simulink model "systemmain"  (R2017b)
settings: Solver=VariableStepAuto  StartTime=0.0  StopTime=20  RelTol=1e-3
values from neighbouring files (symbols this model uses):
  Kd_alt = 0    [Controller_Tuning.m]
  Kd_pitch = 0    [Controller_Tuning.m]
  Kd_roll = 0    [Controller_Tuning.m]
  Kd_yaw = 0    [Controller_Tuning.m]
  Ki_alt = 0    [Controller_Tuning.m]
  Ki_pitch = 1    [Controller_Tuning.m]
  Ki_roll = 1    [Controller_Tuning.m]
  Ki_yaw = 1    [Controller_Tuning.m]
  Kp_alt = 1    [Controller_Tuning.m]
  Kp_pitch = 1    [Controller_Tuning.m]
  Kp_roll = 1    [Controller_Tuning.m]
  Kp_yaw = 1    [Controller_Tuning.m]
  phiaccinitial = 0    [startup.m]
  phiinitial = 0    [startup.m]
  phivelinitial = 0    [startup.m]
  psiaccinitial = 0    [startup.m]
  psiinitial = 0    [startup.m]
  psivelinitial = 0    [startup.m]
  thetaaccinitial = 0    [startup.m]
  thetainitial = 0    [startup.m]
  thetavelinitial = 0    [startup.m]
  xaccinitial = 0    [startup.m]
  xinitial = 0    [startup.m]
  xvelinitial = 0    [startup.m]
  yaccinitial = 0    [startup.m]
  yinitial = 0    [startup.m]
  yvelinitial = 0    [startup.m]
  zaccinitial = 0    [startup.m]
  zinitial = 10    [startup.m]
  zvelinitial = 0    [startup.m]
libraries: simulink x4
settings Model: Creator=DanAdmin  LastModifiedBy=schapman

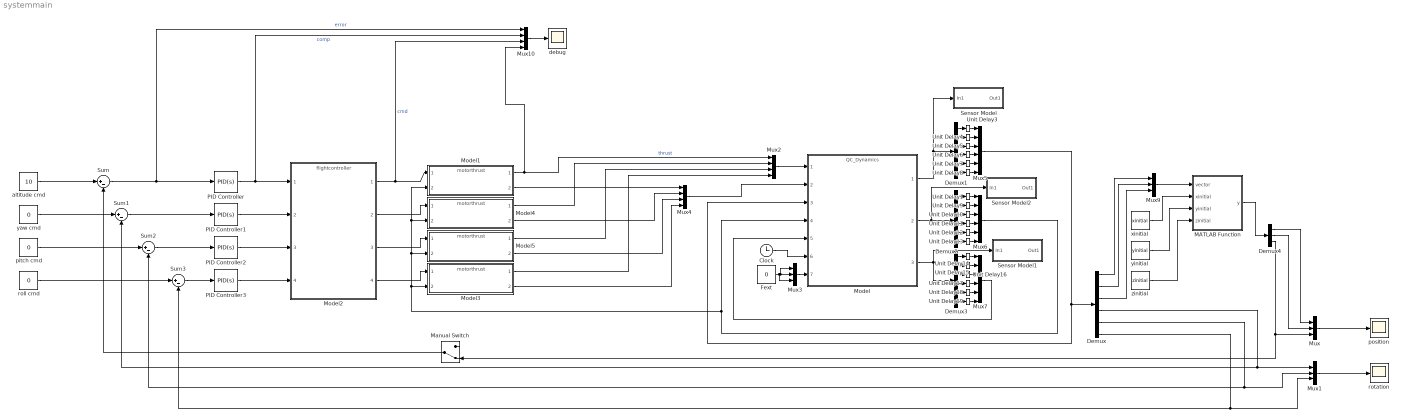
== system systemmain ==
  Clock : Clock
  Demux{,1..3} (4 alike) : Demux  Outputs=6
  Demux4 : Demux  Outputs=3
  Fext : Constant  Value=0
  MATLAB Function : MATLAB Function  TreatAsAtomicUnit=on
  Manual Switch : ManualSwitch  CurrentSetting=0
  Model : ModelReference  ModelNameDialog=QC_Dynamics  SimulationMode=Normal  ModelReferenceVersion=1.26
  Model{1,3..5} (4 alike) : ModelReference  ModelNameDialog=motorthrust  SimulationMode=Normal  ModelReferenceVersion=1.24
  Model2 : ModelReference  ModelNameDialog=flightcontroller.slx  SimulationMode=Normal  ModelReferenceVersion=1.13
  Mux{,1,3,9} (4 alike) : Mux  Inputs=3
  Mux10 : Mux
  Mux2 : Mux
  Mux4 : Mux
  Mux5 : Mux  Inputs=6
  Mux6 : Mux  Inputs=6
  Mux7 : Mux  Inputs=6
  PID Controller : simulink/Continuous/PID Controller  Controller=PID  TimeDomain=Continuous-time  SampleTime=-1  IntegratorMethod=Forward Euler  FilterMethod=Forward Euler  Form=Parallel  UseFilter=on  ControllerParametersSource=internal  P=Kp_alt  I=Ki_alt  D=Kd_alt  N=100  InitialConditionSource=internal  InitialConditionForIntegrator=0  InitialConditionForFilter=0  ExternalReset=none  LimitOutput=off  UpperSaturationLimit=inf  LowerSaturationLimit=-inf  LinearizeAsGain=on  AntiWindupMode=none  Kb=1  TrackingMode=off  Kt=1  PParamMin=[]  PParamMax=[]  IParamMin=[]  IParamMax=[]  DParamMin=[]  DParamMax=[]  NParamMin=[]  NParamMax=[]  KbParamMin=[]  KbParamMax=[]  KtParamMin=[]  KtParamMax=[]  POutMin=[]  POutMax=[]  IOutMin=[]  IOutMax=[]  DOutMin=[]  DOutMax=[]  NOutMin=[]  NOutMax=[]  KbOutMin=[]  KbOutMax=[]  KtOutMin=[]  KtOutMax=[]  IntegratorOutMin=[]  IntegratorOutMax=[]  FilterOutMin=[]  FilterOutMax=[]  SumOutMin=[]  SumOutMax=[]  SumI1OutMin=[]  SumI1OutMax=[]  SumI2OutMin=[]  SumI2OutMax=[]  SumI3OutMin=[]  SumI3OutMax=[]  SumDOutMin=[]  SumDOutMax=[]  SaturationOutMin=[]  SaturationOutMax=[]  IntegratorContinuousStateAttributes=''  IntegratorStateMustResolveToSignalObject=off  IntegratorRTWStateStorageClass=Auto  FilterContinuousStateAttributes=''  FilterStateMustResolveToSignalObject=off  FilterRTWStateStorageClass=Auto  DifferentiatorICPrevScaledInput=0  DifferentiatorOutMin=[]  DifferentiatorOutMax=[]  InitialConditionSetting=State (most efficient)  FilterDiffOutCoefMin=[]  FilterDiffOutCoefMax=[]  SumDenOutMin=[]  SumDenOutMax=[]  SumNumOutMin=[]  SumNumOutMax=[]  ReciprocalOutMin=[]  ReciprocalOutMax=[]  DivideOutMin=[]  DivideOutMax=[]  TunerSelectOption=Transfer Function Based (PID Tuner App)
  PID Controller1 : simulink/Continuous/PID Controller  Controller=PID  TimeDomain=Continuous-time  SampleTime=-1  IntegratorMethod=Forward Euler  FilterMethod=Forward Euler  Form=Parallel  UseFilter=on  ControllerParametersSource=internal  P=Kp_yaw  I=Ki_yaw  D=Kd_yaw  N=100  InitialConditionSource=internal  InitialConditionForIntegrator=0  InitialConditionForFilter=0  ExternalReset=none  LimitOutput=off  UpperSaturationLimit=inf  LowerSaturationLimit=-inf  LinearizeAsGain=on  AntiWindupMode=none  Kb=1  TrackingMode=off  Kt=1  PParamMin=[]  PParamMax=[]  IParamMin=[]  IParamMax=[]  DParamMin=[]  DParamMax=[]  NParamMin=[]  NParamMax=[]  KbParamMin=[]  KbParamMax=[]  KtParamMin=[]  KtParamMax=[]  POutMin=[]  POutMax=[]  IOutMin=[]  IOutMax=[]  DOutMin=[]  DOutMax=[]  NOutMin=[]  NOutMax=[]  KbOutMin=[]  KbOutMax=[]  KtOutMin=[]  KtOutMax=[]  IntegratorOutMin=[]  IntegratorOutMax=[]  FilterOutMin=[]  FilterOutMax=[]  SumOutMin=[]  SumOutMax=[]  SumI1OutMin=[]  SumI1OutMax=[]  SumI2OutMin=[]  SumI2OutMax=[]  SumI3OutMin=[]  SumI3OutMax=[]  SumDOutMin=[]  SumDOutMax=[]  SaturationOutMin=[]  SaturationOutMax=[]  IntegratorContinuousStateAttributes=''  IntegratorStateMustResolveToSignalObject=off  IntegratorRTWStateStorageClass=Auto  FilterContinuousStateAttributes=''  FilterStateMustResolveToSignalObject=off  FilterRTWStateStorageClass=Auto  DifferentiatorICPrevScaledInput=0  DifferentiatorOutMin=[]  DifferentiatorOutMax=[]  InitialConditionSetting=State (most efficient)  FilterDiffOutCoefMin=[]  FilterDiffOutCoefMax=[]  SumDenOutMin=[]  SumDenOutMax=[]  SumNumOutMin=[]  SumNumOutMax=[]  ReciprocalOutMin=[]  ReciprocalOutMax=[]  DivideOutMin=[]  DivideOutMax=[]  TunerSelectOption=Transfer Function Based (PID Tuner App)
  PID Controller2 : simulink/Continuous/PID Controller  Controller=PID  TimeDomain=Continuous-time  SampleTime=-1  IntegratorMethod=Forward Euler  FilterMethod=Forward Euler  Form=Parallel  UseFilter=on  ControllerParametersSource=internal  P=Kp_pitch  I=Ki_pitch  D=Kd_pitch  N=100  InitialConditionSource=internal  InitialConditionForIntegrator=0  InitialConditionForFilter=0  ExternalReset=none  LimitOutput=off  UpperSaturationLimit=inf  LowerSaturationLimit=-inf  LinearizeAsGain=on  AntiWindupMode=none  Kb=1  TrackingMode=off  Kt=1  PParamMin=[]  PParamMax=[]  IParamMin=[]  IParamMax=[]  DParamMin=[]  DParamMax=[]  NParamMin=[]  NParamMax=[]  KbParamMin=[]  KbParamMax=[]  KtParamMin=[]  KtParamMax=[]  POutMin=[]  POutMax=[]  IOutMin=[]  IOutMax=[]  DOutMin=[]  DOutMax=[]  NOutMin=[]  NOutMax=[]  KbOutMin=[]  KbOutMax=[]  KtOutMin=[]  KtOutMax=[]  IntegratorOutMin=[]  IntegratorOutMax=[]  FilterOutMin=[]  FilterOutMax=[]  SumOutMin=[]  SumOutMax=[]  SumI1OutMin=[]  SumI1OutMax=[]  SumI2OutMin=[]  SumI2OutMax=[]  SumI3OutMin=[]  SumI3OutMax=[]  SumDOutMin=[]  SumDOutMax=[]  SaturationOutMin=[]  SaturationOutMax=[]  IntegratorContinuousStateAttributes=''  IntegratorStateMustResolveToSignalObject=off  IntegratorRTWStateStorageClass=Auto  FilterContinuousStateAttributes=''  FilterStateMustResolveToSignalObject=off  FilterRTWStateStorageClass=Auto  DifferentiatorICPrevScaledInput=0  DifferentiatorOutMin=[]  DifferentiatorOutMax=[]  InitialConditionSetting=State (most efficient)  FilterDiffOutCoefMin=[]  FilterDiffOutCoefMax=[]  SumDenOutMin=[]  SumDenOutMax=[]  SumNumOutMin=[]  SumNumOutMax=[]  ReciprocalOutMin=[]  ReciprocalOutMax=[]  DivideOutMin=[]  DivideOutMax=[]  TunerSelectOption=Transfer Function Based (PID Tuner App)
  PID Controller3 : simulink/Continuous/PID Controller  Controller=PID  TimeDomain=Continuous-time  SampleTime=-1  IntegratorMethod=Forward Euler  FilterMethod=Forward Euler  Form=Parallel  UseFilter=on  ControllerParametersSource=internal  P=Kp_roll  I=Ki_roll  D=Kd_roll  N=100  InitialConditionSource=internal  InitialConditionForIntegrator=0  InitialConditionForFilter=0  ExternalReset=none  LimitOutput=off  UpperSaturationLimit=inf  LowerSaturationLimit=-inf  LinearizeAsGain=on  AntiWindupMode=none  Kb=1  TrackingMode=off  Kt=1  PParamMin=[]  PParamMax=[]  IParamMin=[]  IParamMax=[]  DParamMin=[]  DParamMax=[]  NParamMin=[]  NParamMax=[]  KbParamMin=[]  KbParamMax=[]  KtParamMin=[]  KtParamMax=[]  POutMin=[]  POutMax=[]  IOutMin=[]  IOutMax=[]  DOutMin=[]  DOutMax=[]  NOutMin=[]  NOutMax=[]  KbOutMin=[]  KbOutMax=[]  KtOutMin=[]  KtOutMax=[]  IntegratorOutMin=[]  IntegratorOutMax=[]  FilterOutMin=[]  FilterOutMax=[]  SumOutMin=[]  SumOutMax=[]  SumI1OutMin=[]  SumI1OutMax=[]  SumI2OutMin=[]  SumI2OutMax=[]  SumI3OutMin=[]  SumI3OutMax=[]  SumDOutMin=[]  SumDOutMax=[]  SaturationOutMin=[]  SaturationOutMax=[]  IntegratorContinuousStateAttributes=''  IntegratorStateMustResolveToSignalObject=off  IntegratorRTWStateStorageClass=Auto  FilterContinuousStateAttributes=''  FilterStateMustResolveToSignalObject=off  FilterRTWStateStorageClass=Auto  DifferentiatorICPrevScaledInput=0  DifferentiatorOutMin=[]  DifferentiatorOutMax=[]  InitialConditionSetting=State (most efficient)  FilterDiffOutCoefMin=[]  FilterDiffOutCoefMax=[]  SumDenOutMin=[]  SumDenOutMax=[]  SumNumOutMin=[]  SumNumOutMax=[]  ReciprocalOutMin=[]  ReciprocalOutMax=[]  DivideOutMin=[]  DivideOutMax=[]  TunerSelectOption=Transfer Function Based (PID Tuner App)
  Sensor Model : Subsystem
  Sensor Model1 : Subsystem
  Sensor Model2 : Subsystem
  Sum{,1..3} (4 alike) : Sum  Inputs=|+-
  Unit Delay1 : UnitDelay  InitialCondition=xvelinitial  SampleTime=-1
  Unit Delay10 : UnitDelay  InitialCondition=zvelinitial  SampleTime=-1
  Unit Delay11 : UnitDelay  InitialCondition=phivelinitial  SampleTime=-1
  Unit Delay12 : UnitDelay  InitialCondition=thetavelinitial  SampleTime=-1
  Unit Delay13 : UnitDelay  InitialCondition=psivelinitial  SampleTime=-1
  Unit Delay14 : UnitDelay  InitialCondition=xaccinitial  SampleTime=-1
  Unit Delay15 : UnitDelay  InitialCondition=yaccinitial  SampleTime=-1
  Unit Delay16 : UnitDelay  InitialCondition=zaccinitial  SampleTime=-1
  Unit Delay17 : UnitDelay  InitialCondition=phiaccinitial  SampleTime=-1
  Unit Delay18 : UnitDelay  InitialCondition=thetaaccinitial  SampleTime=-1
  Unit Delay19 : UnitDelay  InitialCondition=psiaccinitial  SampleTime=-1
  Unit Delay3 : UnitDelay  SampleTime=-1
  Unit Delay4 : UnitDelay  SampleTime=-1
  Unit Delay5 : UnitDelay  SampleTime=-1
  Unit Delay6 : UnitDelay  InitialCondition=phiinitial  SampleTime=-1
  Unit Delay7 : UnitDelay  InitialCondition=thetainitial  SampleTime=-1
  Unit Delay8 : UnitDelay  InitialCondition=psiinitial  SampleTime=-1
  Unit Delay9 : UnitDelay  InitialCondition=yvelinitial  SampleTime=-1
  altitude cmd : Constant  Value=10
  debug : Scope
  pitch cmd : Constant  Value=0
  "position " : Scope
  roll cmd : Constant  Value=0
  rotation : Scope
  xinitial : Constant  Value=xinitial
  yaw cmd : Constant  Value=0
  yinitial : Constant  Value=yinitial
  zinitial : Constant  Value=zinitial
  wires:
  PID Controller3/1 -> Model2/4
  PID Controller/1 -> Mux10/2, Model2/1  "comp"
  PID Controller2/1 -> Model2/3
  PID Controller1/1 -> Model2/2
  Model2/1 -> Mux10/3, Model1/1  "cmd"
  Model2/2 -> Model4/1
  Model2/3 -> Model5/1
  Model2/4 -> Model3/1
  Sum/1 -> Mux10/1, PID Controller/1  "error"
  Sum3/1 -> PID Controller3/1
  Sum2/1 -> PID Controller2/1
  Sum1/1 -> PID Controller1/1
  Demux/4 -> Mux1/1, Sum1/2
  Demux/5 -> Sum2/2, Mux1/2
  Demux/6 -> Sum3/2, Mux1/3
  Demux/3 -> Mux9/3
  roll cmd/1 -> Sum3/1
  pitch cmd/1 -> Sum2/1
  yaw cmd/1 -> Sum1/1
  altitude cmd/1 -> Sum/1
  Mux1/1 -> rotation/1
  Demux/1 -> Mux9/1
  Demux/2 -> Mux9/2
  Clock/1 -> Model/6
  Mux3/1 -> Model/7
  Fext/1 -> Mux3/1, Mux3/2, Mux3/3
  Model/1 -> Demux1/1, Sensor Model/1(In1)
  Model/2 -> Demux2/1, Sensor Model2/1(In1)
  Model/3 -> Demux3/1, Sensor Model1/1(In1)
  Mux7/1 -> Model/5
  Mux6/1 -> Model3/2, Model4/2, Model1/2, Model5/2, Model/4
  Mux5/1 -> Model/3, Demux/1
  Mux2/1 -> Model/1
  Model1/1 -> Mux2/1, Mux10/4  "thrust"
  Model4/1 -> Mux2/2
  Model5/1 -> Mux2/3
  Model3/1 -> Mux2/4
  Mux4/1 -> Model/2
  Model1/2 -> Mux4/1
  Model4/2 -> Mux4/2
  Model5/2 -> Mux4/3
  Model3/2 -> Mux4/4
  Manual Switch/1 -> Sum/2
  Unit Delay3/1 -> Mux5/1
  Demux1/1 -> Unit Delay3/1
  Demux1/2 -> Unit Delay4/1
  Unit Delay4/1 -> Mux5/2
  Demux1/3 -> Unit Delay5/1
  Unit Delay5/1 -> Mux5/3
  Demux1/4 -> Unit Delay6/1
  Unit Delay6/1 -> Mux5/4
  Demux1/5 -> Unit Delay7/1
  Unit Delay7/1 -> Mux5/5
  Demux1/6 -> Unit Delay8/1
  Unit Delay8/1 -> Mux5/6
  Unit Delay9/1 -> Mux6/2
  Unit Delay1/1 -> Mux6/1
  Unit Delay11/1 -> Mux6/4
  Unit Delay10/1 -> Mux6/3
  Demux2/3 -> Unit Delay10/1
  Demux2/1 -> Unit Delay1/1
  Unit Delay12/1 -> Mux6/5
  Demux2/6 -> Unit Delay13/1
  Demux2/5 -> Unit Delay12/1
  Demux2/4 -> Unit Delay11/1
  Demux2/2 -> Unit Delay9/1
  Unit Delay13/1 -> Mux6/6
  Unit Delay15/1 -> Mux7/2
  Unit Delay14/1 -> Mux7/1
  Unit Delay17/1 -> Mux7/4
  Unit Delay16/1 -> Mux7/3
  Demux3/3 -> Unit Delay16/1
  Demux3/1 -> Unit Delay14/1
  Unit Delay18/1 -> Mux7/5
  Demux3/6 -> Unit Delay19/1
  Demux3/5 -> Unit Delay18/1
  Demux3/4 -> Unit Delay17/1
  Demux3/2 -> Unit Delay15/1
  Unit Delay19/1 -> Mux7/6
  Mux/1 -> "position "/1
  Mux9/1 -> MATLAB Function/1(vector)
  Demux4/1 -> Mux/1
  Demux4/2 -> Mux/2
  Demux4/3 -> Manual Switch/2, Mux/3
  Mux10/1 -> debug/1
  MATLAB Function/1(y) -> Demux4/1
  xinitial/1 -> MATLAB Function/2(xinitial)
  yinitial/1 -> MATLAB Function/3(yinitial)
  zinitial/1 -> MATLAB Function/4(zinitial)

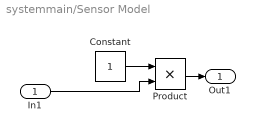
== system systemmain/Sensor Model ==
  In1 : Inport
  Constant : Constant
  Product : Product
  Out1 : Outport
  wires:
  Constant/1 -> Product/1
  Product/1 -> Out1/1
  In1/1 -> Product/2

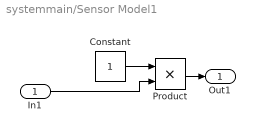
== system systemmain/Sensor Model1 ==
  In1 : Inport
  Constant : Constant
  Product : Product
  Out1 : Outport
  wires:
  Constant/1 -> Product/1
  Product/1 -> Out1/1
  In1/1 -> Product/2

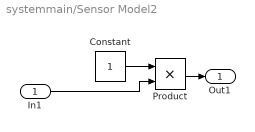
== system systemmain/Sensor Model2 ==
  In1 : Inport
  Constant : Constant
  Product : Product
  Out1 : Outport
  wires:
  Constant/1 -> Product/1
  Product/1 -> Out1/1
  In1/1 -> Product/2

== matlab function systemmain/MATLAB Function ==
  data: vector input; y output; xinitial input; yinitial input; zinitial input
function y = fcn(vector, xinitial, yinitial, zinitial)

rot=[pi,0,0];

%R=[1,0,0;0,cos(rot(1)),-sin(rot(1));0,sin(rot(1)),cos(rot(1))]*[cos(rot(2)),0, -sin(rot(2));0,1,0;sin(rot(2)),0,cos(rot(2))]*[cos(rot(3)),-sin(rot(3)),0;sin(rot(3)),cos(rot(3)),0;0,0,1];

Rx=[1,0,0;0,cos(rot(1)),-sin(rot(1));0,sin(rot(1)),cos(rot(1))];
Ry=[cos(rot(2)),0, sin(rot(2));0,1,0;-sin(rot(2)),0,cos(rot(2))];
Rz=[cos(rot(3)),-sin(rot(3)),0;sin(rot(3)),cos(rot(3)),0;0,0,1];

R=Rx;


w=R*vector
y=w+[xinitial;yinitial;zinitial];
end
